simulink model "task2"  (R2016b)
settings: Solver=VariableStepAuto  StartTime=0.0  StopTime=10.0  RelTol=1e-3
libraries: commutil2 x2
settings Model: Creator=zhangjin  LastModifiedBy=zhangjin

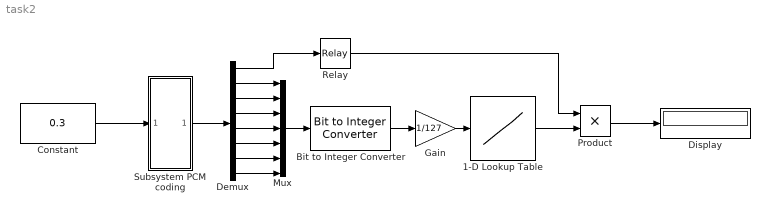
== system task2 ==
  1-D Lookup Table : Lookup_n-D  NumberOfTableDimensions=1  BreakpointsForDimension1=[-5:5]  Table=tanh([-5:5])  InternalRulePriority=Speed  RndMeth=Simplest  InputSameDT=on
  Bit to Integer Converter : commutil2/Bit to Integer Converter  nbits=3  bitOrder=MSB first  signedOutputValues=Unsigned  outDtype=Inherit via internal rule  outDtypeSigned=Inherit via internal rule
  Constant : Constant  Value=0.3
  Demux : Demux  Outputs=8
  Display : Display
  Gain : Gain  Gain=1/127
  Mux : Mux  Inputs=7
  Product : Product
  Relay : Relay
  Subsystem PCM coding : Subsystem
  wires:
  Constant/1 -> Subsystem PCM coding/1(In1)
  Subsystem PCM coding/1(Out1) -> Demux/1
  Demux/1 -> Relay/1
  Demux/2 -> Mux/1
  Demux/3 -> Mux/2
  Demux/4 -> Mux/3
  Demux/5 -> Mux/4
  Demux/6 -> Mux/5
  Demux/7 -> Mux/6
  Demux/8 -> Mux/7
  Mux/1 -> Bit to Integer Converter/1
  Bit to Integer Converter/1 -> Gain/1
  Gain/1 -> 1-D Lookup Table/1
  1-D Lookup Table/1 -> Product/2
  Relay/1 -> Product/1
  Product/1 -> Display/1

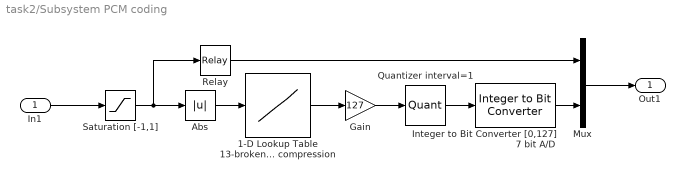
== system task2/Subsystem PCM coding ==
  In1 : Inport
  1-D Lookup Table 13-broken line compression : Lookup_n-D  NumberOfTableDimensions=1  BreakpointsForDimension1=[-5:5]  Table=tanh([-5:5])  InternalRulePriority=Speed  RndMeth=Simplest  InputSameDT=on
  Abs : Abs
  Gain : Gain  Gain=127
  Integer to Bit Converter [0,127] 7 bit A/D : commutil2/Integer to Bit Converter  nbits=3  signedInputValues=Unsigned  bitOrder=MSB first  outDtype=Inherit via internal rule
  Mux : Mux  Inputs=2
  Quantizer interval=1 : Quantizer  QuantizationInterval=1  LinearizeAsGain=off
  Relay : Relay
  Saturation [-1,1] : Saturate  UpperLimit=1  LowerLimit=-1
  Out1 : Outport
  wires:
  In1/1 -> Saturation [-1,1]/1
  Saturation [-1,1]/1 -> Relay/1, Abs/1
  Abs/1 -> 1-D Lookup Table 13-broken line compression/1
  1-D Lookup Table 13-broken line compression/1 -> Gain/1
  Gain/1 -> Quantizer interval=1/1
  Quantizer interval=1/1 -> Integer to Bit Converter [0,127] 7 bit A/D/1
  Integer to Bit Converter [0,127] 7 bit A/D/1 -> Mux/2
  Relay/1 -> Mux/1
  Mux/1 -> Out1/1
